simulink model "vtol_roll_kin"  (R2021a)
settings: Solver=VariableStepAuto  StartTime=0.0  StopTime=60  RelTol=1e-8
undefined symbols (not defined in the file): Ckf, cphi, cy, cz, disturbance_on, g, Jxx, Klqr, ky, kz, l, m, noise_on, phidote, phie, sysKF, u1e, Vwind_ll, Vwind_ul, ydote, ye, zdote, ze
libraries: aerolibwind2 x1
settings Model: Creator=Tomo  LastModifiedBy=Tomo

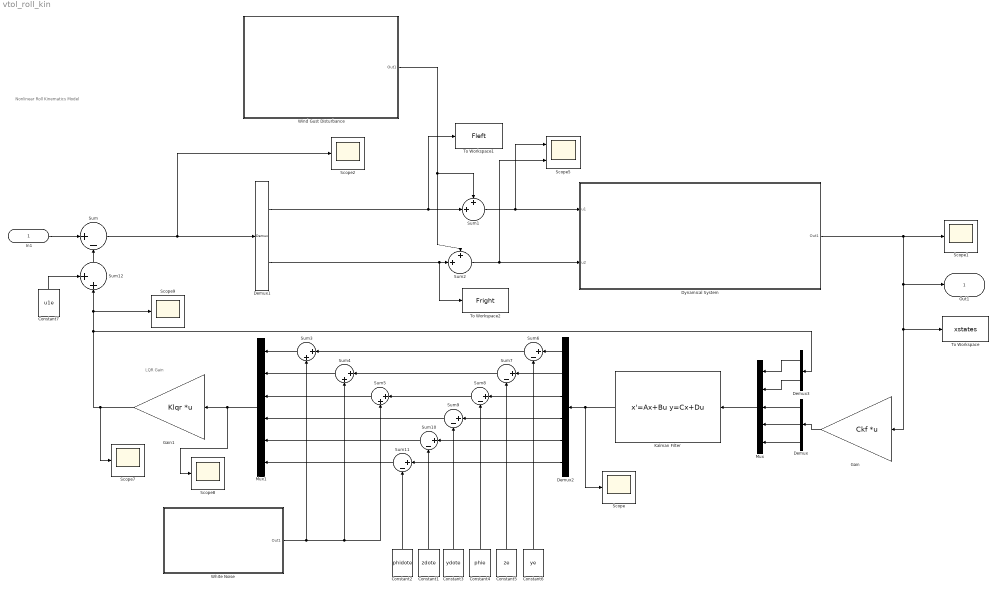
== system vtol_roll_kin ==
  note: LQR Gain
  note: Nonlinear Roll Kinematics Model
  In1 : Inport
  Constant1 : Constant  Value=zdote
  Constant2 : Constant  Value=phidote
  Constant3 : Constant  Value=ydote
  Constant4 : Constant  Value=phie
  Constant5 : Constant  Value=ze
  Constant6 : Constant  Value=ye
  Constant7 : Constant  Value=u1e
  Demux : Demux  Outputs=3
  Demux1 : Demux  Outputs=2
  Demux2 : Demux  Outputs=6
  Demux3 : Demux  Outputs=2
  Dynamical System : Subsystem
  Gain : Gain  Gain=Ckf  Multiplication=Matrix(K*u)
  Gain1 : Gain  Gain=Klqr  Multiplication=Matrix(K*u)
  Kalman Filter : StateSpace  A=sysKF.A  B=sysKF.B  C=sysKF.C  D=sysKF.D  InitialCondition=[ye ze phie ydote zdote phidote]
  Mux : Mux  Inputs=5
  Mux1 : Mux  Inputs=6
  Scope{,1..2,7..9} (6 alike) : Scope
  Scope5 : Scope  NumInputPorts=2
  Sum{,6..11} (7 alike) : Sum  Inputs=|+-
  Sum1 : Sum  Inputs=++|
  Sum12 : Sum  Inputs=++|
  Sum2 : Sum  Inputs=++|
  Sum3 : Sum  Inputs=|++
  Sum4 : Sum  Inputs=|++
  Sum5 : Sum  Inputs=|++
  To Workspace : ToWorkspace  VariableName=xstates  SaveFormat=Structure With Time  SampleTime=-1
  To Workspace1 : ToWorkspace  VariableName=Fleft  SaveFormat=Structure With Time  SampleTime=-1
  To Workspace2 : ToWorkspace  VariableName=Fright  SaveFormat=Structure With Time  SampleTime=-1
  White Noise : Subsystem
  Wind Gust Disturbance : Subsystem
  Out1 : Outport
  wires:
  Mux/1 -> Kalman Filter/1
  Mux1/1 -> Scope8/1, Gain1/1
  Kalman Filter/1 -> Scope/1, Demux2/1
  Demux2/4 -> Sum9/1
  Demux2/5 -> Sum10/1
  Demux2/6 -> Sum11/1
  Demux2/1 -> Sum6/1
  Sum3/1 -> Mux1/1
  Sum4/1 -> Mux1/2
  Demux2/2 -> Sum7/1
  Demux2/3 -> Sum8/1
  Sum5/1 -> Mux1/3
  White Noise/1(Out1) -> Sum3/2, Sum5/2, Sum4/2
  Sum6/1 -> Sum3/1
  Sum7/1 -> Sum4/1
  Sum8/1 -> Sum5/1
  Sum9/1 -> Mux1/4
  Sum10/1 -> Mux1/5
  Sum11/1 -> Mux1/6
  Constant2/1 -> Sum11/2
  Constant1/1 -> Sum10/2
  Constant3/1 -> Sum9/2
  Constant4/1 -> Sum8/2
  Constant5/1 -> Sum7/2
  Constant6/1 -> Sum6/2
  In1/1 -> Sum/1
  Dynamical System/1(Out1) -> Out1/1, Gain/1, To Workspace/1, Scope1/1
  Gain/1 -> Demux/1
  Demux/2 -> Mux/4
  Demux3/1 -> Mux/1
  Demux3/2 -> Mux/2
  Wind Gust Disturbance/1(Out1) -> Sum1/1, Sum2/1
  Sum1/1 -> Scope5/1, Dynamical System/1(u1)
  Sum2/1 -> Scope5/2, Dynamical System/2(u2)
  Demux/3 -> Mux/5
  Demux/1 -> Mux/3
  Sum/1 -> Scope2/1, Demux1/1
  Demux1/2 -> To Workspace2/1, Sum2/2
  Demux1/1 -> To Workspace1/1, Sum1/2
  Gain1/1 -> Sum12/2, Scope9/1, Demux3/1, Scope7/1
  Constant7/1 -> Sum12/1
  Sum12/1 -> Sum/2

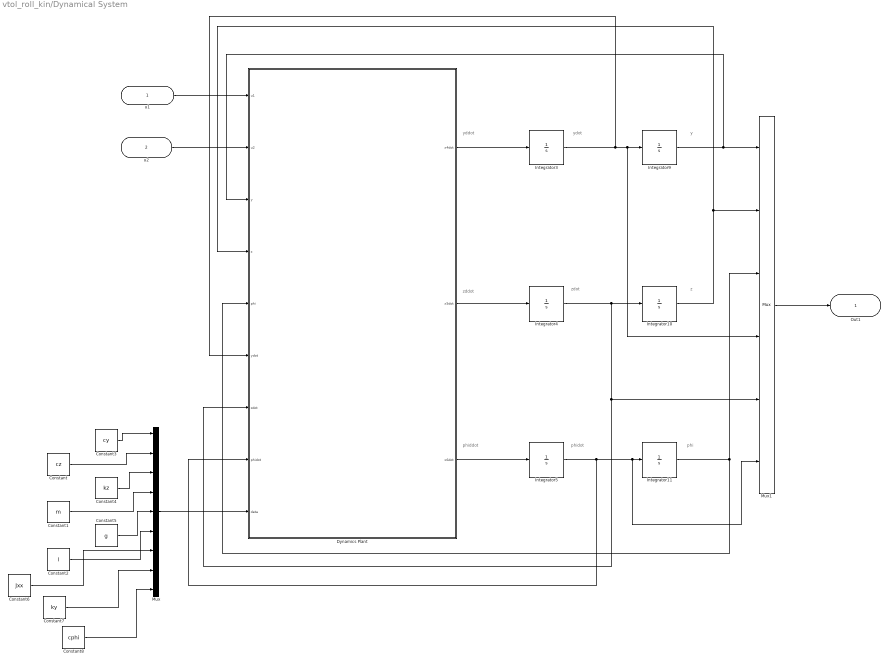
== system vtol_roll_kin/Dynamical System ==
  note: phiddot
  note: yddot
  note: zddot
  note: y
  note: z
  note: phi
  note: ydot
  note: zdot
  note: phidot
  u1 : Inport
  u2 : Inport  Port=2
  Constant : Constant  Value=cz
  Constant1 : Constant  Value=m
  Constant2 : Constant  Value=l
  Constant3 : Constant  Value=cy
  Constant4 : Constant  Value=kz
  Constant5 : Constant  Value=g
  Constant6 : Constant  Value=Jxx
  Constant7 : Constant  Value=ky
  Constant8 : Constant  Value=cphi
  Dynamics Plant : MATLAB Function  TreatAsAtomicUnit=on
  Integrator{3..5,9..11} (6 alike) : Integrator
  Mux : Mux  Inputs=9
  Mux1 : Mux  Inputs=6
  Out1 : Outport
  wires:
  Constant1/1 -> Mux/4
  Constant5/1 -> Mux/5
  Integrator3/1 -> Dynamics Plant/6(ydot), Mux1/4, Integrator9/1
  Integrator10/1 -> Dynamics Plant/4(z), Mux1/2
  Integrator5/1 -> Dynamics Plant/8(phidot), Mux1/6, Integrator11/1
  Integrator9/1 -> Dynamics Plant/3(y), Mux1/1
  Constant6/1 -> Mux/7
  Integrator4/1 -> Dynamics Plant/7(zdot), Mux1/5, Integrator10/1
  Constant2/1 -> Mux/6
  Dynamics Plant/1(x4dot) -> Integrator3/1
  Mux/1 -> Dynamics Plant/9(data)
  u1/1 -> Dynamics Plant/1(u1)
  Dynamics Plant/3(x6dot) -> Integrator5/1
  Integrator11/1 -> Mux1/3, Dynamics Plant/5(phi)
  u2/1 -> Dynamics Plant/2(u2)
  Dynamics Plant/2(x5dot) -> Integrator4/1
  Constant3/1 -> Mux/1
  Constant4/1 -> Mux/3
  Constant/1 -> Mux/2
  Mux1/1 -> Out1/1
  Constant7/1 -> Mux/8
  Constant8/1 -> Mux/9

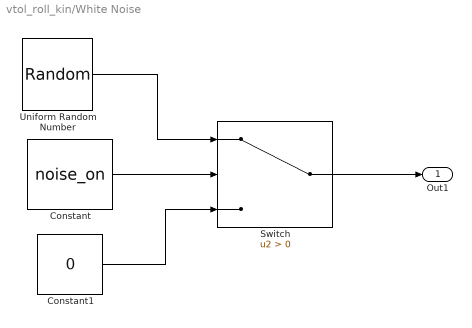
== system vtol_roll_kin/White Noise ==
  Constant : Constant  Value=noise_on
  Constant1 : Constant  Value=0
  Switch : Switch  Criteria=u2 > Threshold
  Uniform Random Number : UniformRandomNumber  Minimum=-0.1  Maximum=0.1  SampleTime=0.1
  Out1 : Outport
  wires:
  Constant/1 -> Switch/2
  Constant1/1 -> Switch/3
  Uniform Random Number/1 -> Switch/1
  Switch/1 -> Out1/1

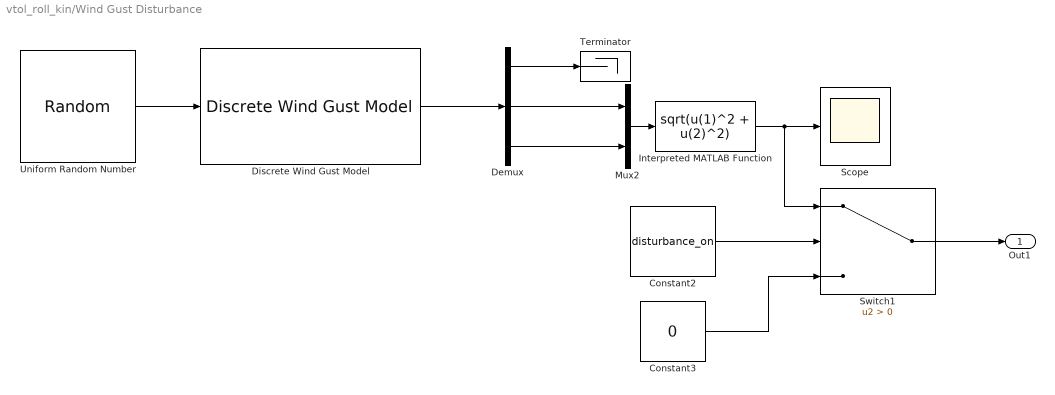
== system vtol_roll_kin/Wind Gust Disturbance ==
  Constant2 : Constant  Value=disturbance_on
  Constant3 : Constant  Value=0
  Demux : Demux  Outputs=3
  Discrete Wind Gust Model : aerolibwind2/Discrete Wind Gust Model  units=Metric (MKS)  Gx=off  Gy=on  Gz=on  t_0=6  d_m=[120 120 80]  v_m=[23 23 23]
  Interpreted MATLAB Function : MATLABFcn  MATLABFcn=sqrt(u(1)^2 + u(2)^2)
  Mux2 : Mux  Inputs=2
  Scope : Scope
  Switch1 : Switch  Criteria=u2 > Threshold
  Terminator : Terminator
  Uniform Random Number : UniformRandomNumber  Minimum=Vwind_ll  Maximum=Vwind_ul  Seed=1  SampleTime=0.65
  Out1 : Outport
  wires:
  Interpreted MATLAB Function/1 -> Switch1/1, Scope/1
  Demux/1 -> Terminator/1
  Mux2/1 -> Interpreted MATLAB Function/1
  Discrete Wind Gust Model/1 -> Demux/1
  Demux/2 -> Mux2/1
  Uniform Random Number/1 -> Discrete Wind Gust Model/1
  Constant2/1 -> Switch1/2
  Constant3/1 -> Switch1/3
  Demux/3 -> Mux2/2
  Switch1/1 -> Out1/1

== matlab function vtol_roll_kin/Dynamical System/Dynamics Plant ==
  data: u1 input; u2 input; y input; z input; phi input; ydot input; zdot input; phidot input; x4dot output; x5dot output; x6dot output; data input
function [x4dot, x5dot, x6dot] = fcn(u1, u2, y, z, phi, ydot, zdot, phidot, data)
    % Constants
    cy   = data(1);
    cz   = data(2);
    kz   = data(3);
    m    = data(4);
    g    = data(5);
    l    = data(6);
    Jxx  = data(7);
    ky   = data(8);
    cphi = data(9);
    
    % ydot = x1dot, zdot = x2dot, phidot = x3dot
    % yddot = x4dot, zddot = x5dot, phiddot = x6dot
    
    x4dot = -ky/m*y - cy/m*ydot + u1*sin(phi)/m + u2*sin(phi)/m;
    x5dot = -kz/m*z - cz/m*zdot - u1*cos(phi)/m - u2*cos(phi)/m + g;
    x6dot = -cphi/Jxx*phidot + l/Jxx*u1 - l/Jxx*u2;
end
